simulink library "halin"  (R2021b)
settings: Solver=VariableStepAuto  StartTime=0.0  StopTime=10.0  RelTol=1e-3
undefined symbols (not defined in the file): TRUE
libraries: FVT_lib x100, hcu_lib x41
(part 9 of 10)

== system halin/HAL_IN/CAN3/MCU_B_R1/RrMCUErr ==
  Rr_MCUErr : Inport
  UnitConverter : DataTypeConversion  OutDataTypeStr=uint8
  VHAL_RrMCUErr_enum : Outport
  wires:
  UnitConverter/1 -> VHAL_RrMCUErr_enum/1
  Rr_MCUErr/1 -> UnitConverter/1

== system halin/HAL_IN/CAN3/MCU_B_R1/RrMCUIGNsta ==
  Rr_MCUIGN_sta : Inport
  UnitConverter : DataTypeConversion  OutDataTypeStr=uint8
  VHAL_RrMCUIGNsta_flg : Outport
  wires:
  UnitConverter/1 -> VHAL_RrMCUIGNsta_flg/1
  Rr_MCUIGN_sta/1 -> UnitConverter/1

== system halin/HAL_IN/CAN3/MCU_B_R1/RrMCUReady ==
  Rr_MCUReady : Inport
  UnitConverter : DataTypeConversion  OutDataTypeStr=uint8
  VHAL_RrMCUReady_flg : Outport
  wires:
  UnitConverter/1 -> VHAL_RrMCUReady_flg/1
  Rr_MCUReady/1 -> UnitConverter/1

== system halin/HAL_IN/CAN3/MCU_B_R1/RrMCUReady4Pre ==
  Rr_MCUReady4Pre : Inport
  UnitConverter : DataTypeConversion  OutDataTypeStr=uint8
  VHAL_RrMCUReady4Pre_flg : Outport
  wires:
  UnitConverter/1 -> VHAL_RrMCUReady4Pre_flg/1
  Rr_MCUReady4Pre/1 -> UnitConverter/1

== system halin/HAL_IN/CAN3/MCU_B_R1/RrMCUSysSta ==
  Rr_MCUSysSta : Inport
  UnitConverter : DataTypeConversion  OutDataTypeStr=uint8
  VHAL_RrMCUSysSta_enum : Outport
  wires:
  UnitConverter/1 -> VHAL_RrMCUSysSta_enum/1
  Rr_MCUSysSta/1 -> UnitConverter/1

== system halin/HAL_IN/CAN3/MCU_B_R1/RrMCUTemp ==
  Rr_MCUTemp : Inport
  UnitConverter : DataTypeConversion  OutDataTypeStr=uint16
  convert_in : FVT_lib/hal/convert_in  gain=1  offset=-40
  VHAL_RrMCUTemp_C : Outport
  wires:
  convert_in/1 -> VHAL_RrMCUTemp_C/1
  UnitConverter/1 -> convert_in/1
  Rr_MCUTemp/1 -> UnitConverter/1

== system halin/HAL_IN/CAN3/MCU_B_R1/RrMotorAvailTq ==
  Rr_MotorAvailTq : Inport
  UnitConverter : DataTypeConversion  OutDataTypeStr=uint16
  VHAL_RrMotorAvailTq_Nm : Outport
  wires:
  UnitConverter/1 -> VHAL_RrMotorAvailTq_Nm/1
  Rr_MotorAvailTq/1 -> UnitConverter/1

== system halin/HAL_IN/CAN3/MCU_B_R1/RrRegenAvailTq ==
  Rr_RegenAvailTq : Inport
  UnitConverter : DataTypeConversion  OutDataTypeStr=uint16
  convert_in : FVT_lib/hal/convert_in  gain=1  offset=-1022
  VHAL_RrRegenAvailTq_Nm : Outport
  wires:
  convert_in/1 -> VHAL_RrRegenAvailTq_Nm/1
  UnitConverter/1 -> convert_in/1
  Rr_RegenAvailTq/1 -> UnitConverter/1

== system halin/HAL_IN/CAN3/MCU_B_R1/RrTMSpd ==
  Rr_TMSpd : Inport
  UnitConverter : DataTypeConversion  OutDataTypeStr=uint16
  convert_in : FVT_lib/hal/convert_in  gain=1  offset=-18000
  VHAL_RrTMSpd_rpm : Outport
  wires:
  convert_in/1 -> VHAL_RrTMSpd_rpm/1
  UnitConverter/1 -> convert_in/1
  Rr_TMSpd/1 -> UnitConverter/1

== system halin/HAL_IN/CAN3/MCU_B_R1/RrTMTemp ==
  Rr_TMTemp : Inport
  UnitConverter : DataTypeConversion  OutDataTypeStr=uint16
  convert_in : FVT_lib/hal/convert_in  gain=1  offset=-40
  VHAL_RrTMTemp_C : Outport
  wires:
  convert_in/1 -> VHAL_RrTMTemp_C/1
  UnitConverter/1 -> convert_in/1
  Rr_TMTemp/1 -> UnitConverter/1

== system halin/HAL_IN/CAN3/MCU_B_R1/RrTMid ==
  Rr_TMid : Inport
  UnitConverter : DataTypeConversion  OutDataTypeStr=uint16
  convert_in : FVT_lib/hal/convert_in  gain=0.1  offset=-1500
  VHAL_RrTMid_A : Outport
  wires:
  convert_in/1 -> VHAL_RrTMid_A/1
  UnitConverter/1 -> convert_in/1
  Rr_TMid/1 -> UnitConverter/1

== system halin/HAL_IN/CAN3/MCU_B_R1/RrTMiq ==
  Rr_TMiq : Inport
  UnitConverter : DataTypeConversion  OutDataTypeStr=uint16
  convert_in : FVT_lib/hal/convert_in  gain=0.1  offset=-1500
  VHAL_RrTMiq_A : Outport
  wires:
  convert_in/1 -> VHAL_RrTMiq_A/1
  UnitConverter/1 -> convert_in/1
  Rr_TMiq/1 -> UnitConverter/1

== system halin/HAL_IN/CAN3/MCU_B_R2/RrCoolanttempReq ==
  Rr_CoolanttempReq : Inport
  UnitConverter : DataTypeConversion  OutDataTypeStr=uint16
  convert_in : FVT_lib/hal/convert_in  gain=1  offset=-40
  VHAL_RrCoolanttempReq_cnt : Outport
  wires:
  convert_in/1 -> VHAL_RrCoolanttempReq_cnt/1
  UnitConverter/1 -> convert_in/1
  Rr_CoolanttempReq/1 -> UnitConverter/1

== system halin/HAL_IN/CAN3/MCU_B_R2/RrFailcode1 ==
  Rr_Failcode1 : Inport
  UnitConverter : DataTypeConversion  OutDataTypeStr=uint8
  VHAL_RrFailcode1_enum : Outport
  wires:
  UnitConverter/1 -> VHAL_RrFailcode1_enum/1
  Rr_Failcode1/1 -> UnitConverter/1

== system halin/HAL_IN/CAN3/MCU_B_R2/RrFailcode2 ==
  Rr_Failcode2 : Inport
  UnitConverter : DataTypeConversion  OutDataTypeStr=uint8
  VHAL_RrFailcode2_enum : Outport
  wires:
  UnitConverter/1 -> VHAL_RrFailcode2_enum/1
  Rr_Failcode2/1 -> UnitConverter/1

== system halin/HAL_IN/CAN3/MCU_B_R2/RrFailcodehistory1 ==
  Rr_Failcodehistory1 : Inport
  UnitConverter : DataTypeConversion  OutDataTypeStr=uint8
  VHAL_RrFailcodehistory1_enum : Outport
  wires:
  UnitConverter/1 -> VHAL_RrFailcodehistory1_enum/1
  Rr_Failcodehistory1/1 -> UnitConverter/1

== system halin/HAL_IN/CAN3/MCU_B_R2/RrFailcodehistory2 ==
  Rr_Failcodehistory2 : Inport
  UnitConverter : DataTypeConversion  OutDataTypeStr=uint8
  VHAL_RrFailcodehistory2_enum : Outport
  wires:
  UnitConverter/1 -> VHAL_RrFailcodehistory2_enum/1
  Rr_Failcodehistory2/1 -> UnitConverter/1

== system halin/HAL_IN/CAN3/MCU_B_R2/RrLLCTemp ==
  Rr_LLCTemp : Inport
  UnitConverter : DataTypeConversion  OutDataTypeStr=uint16
  convert_in : FVT_lib/hal/convert_in  gain=1  offset=-40
  VHAL_RrLLCTemp_C : Outport
  wires:
  convert_in/1 -> VHAL_RrLLCTemp_C/1
  UnitConverter/1 -> convert_in/1
  Rr_LLCTemp/1 -> UnitConverter/1

== system halin/HAL_IN/CAN3/MCU_B_R2/RrLLCflowReq ==
  Rr_LLCflowReq : Inport
  UnitConverter : DataTypeConversion  OutDataTypeStr=uint8
  convert_in : FVT_lib/hal/convert_in  gain=0.25  offset=0
  VHAL_RrLLCflowReq_Lpmin : Outport
  wires:
  convert_in/1 -> VHAL_RrLLCflowReq_Lpmin/1
  UnitConverter/1 -> convert_in/1
  Rr_LLCflowReq/1 -> UnitConverter/1

== system halin/HAL_IN/CAN3/MCU_B_R2/RrMCU3HWVer ==
  Rr_MCU3_HW_Ver : Inport
  UnitConverter : DataTypeConversion  OutDataTypeStr=uint16
  VHAL_RrMCU3HWVer_enum : Outport
  wires:
  UnitConverter/1 -> VHAL_RrMCU3HWVer_enum/1
  Rr_MCU3_HW_Ver/1 -> UnitConverter/1

== system halin/HAL_IN/CAN3/MCU_B_R2/RrMCU3SWVer ==
  Rr_MCU3_SW_Ver : Inport
  UnitConverter : DataTypeConversion  OutDataTypeStr=uint16
  VHAL_RrMCU3SWVer_enum : Outport
  wires:
  UnitConverter/1 -> VHAL_RrMCU3SWVer_enum/1
  Rr_MCU3_SW_Ver/1 -> UnitConverter/1

== system halin/HAL_IN/CAN3/MCU_B_R2/RrMCUTempWarn ==
  Rr_MCUTempWarn : Inport
  UnitConverter : DataTypeConversion  OutDataTypeStr=uint8
  VHAL_RrMCUTempWarn_enum : Outport
  wires:
  UnitConverter/1 -> VHAL_RrMCUTempWarn_enum/1
  Rr_MCUTempWarn/1 -> UnitConverter/1

== system halin/HAL_IN/CAN3/MCU_B_R2/RrTMTempWarn ==
  Rr_TMTempWarn : Inport
  UnitConverter : DataTypeConversion  OutDataTypeStr=uint8
  VHAL_RrTMTempWarn_enum : Outport
  wires:
  UnitConverter/1 -> VHAL_RrTMTempWarn_enum/1
  Rr_TMTempWarn/1 -> UnitConverter/1

== system halin/HAL_IN/CAN3/Shifter1/ShifterCRC8 ==
  Shifter_CRC8 : Inport
  UnitConverter : DataTypeConversion  OutDataTypeStr=uint8
  VHAL_ShifterCRC8_enum : Outport
  wires:
  UnitConverter/1 -> VHAL_ShifterCRC8_enum/1
  Shifter_CRC8/1 -> UnitConverter/1

== system halin/HAL_IN/CAN3/Shifter1/ShifterFailsta ==
  Shifter_Fail_sta : Inport
  UnitConverter : DataTypeConversion  OutDataTypeStr=uint8
  VHAL_ShifterFailsta_enum : Outport
  wires:
  UnitConverter/1 -> VHAL_ShifterFailsta_enum/1
  Shifter_Fail_sta/1 -> UnitConverter/1

== system halin/HAL_IN/CAN3/Shifter1/ShifterHandleCmd ==
  Shifter_Handle_Cmd : Inport
  UnitConverter : DataTypeConversion  OutDataTypeStr=uint8
  VHAL_ShifterHandleCmd_enum : Outport
  wires:
  UnitConverter/1 -> VHAL_ShifterHandleCmd_enum/1
  Shifter_Handle_Cmd/1 -> UnitConverter/1

== system halin/HAL_IN/CAN3/Shifter1/ShifterRC ==
  Shifter_RC : Inport
  UnitConverter : DataTypeConversion  OutDataTypeStr=uint8
  VHAL_ShifterRC_enum : Outport
  wires:
  UnitConverter/1 -> VHAL_ShifterRC_enum/1
  Shifter_RC/1 -> UnitConverter/1

== system halin/HAL_IN/CAN4/DKC1/DKCReVehData ==
  DKC_Re_VehData : Inport
  UnitConverter : DataTypeConversion  OutDataTypeStr=uint8
  VHAL_DKCReVehData_enum : Outport
  wires:
  UnitConverter/1 -> VHAL_DKCReVehData_enum/1
  DKC_Re_VehData/1 -> UnitConverter/1

== system halin/HAL_IN/CAN4/DKC1/PCommandToBCM ==
  P_CommandToBCM : Inport
  UnitConverter : DataTypeConversion  OutDataTypeStr=uint8
  VHAL_PCommandToBCM_enum : Outport
  wires:
  UnitConverter/1 -> VHAL_PCommandToBCM_enum/1
  P_CommandToBCM/1 -> UnitConverter/1

== system halin/HAL_IN/CAN4/DKC1/PCommandToPTG ==
  P_CommandToPTG : Inport
  UnitConverter : DataTypeConversion  OutDataTypeStr=uint8
  VHAL_PCommandToPTG_enum : Outport
  wires:
  UnitConverter/1 -> VHAL_PCommandToPTG_enum/1
  P_CommandToPTG/1 -> UnitConverter/1

== system halin/HAL_IN/CAN4/DKC1/PDKeyAreaLockUnlock ==
  P_DKey_Area_LockUnlock : Inport
  UnitConverter : DataTypeConversion  OutDataTypeStr=uint8
  VHAL_PDKeyAreaLockUnlock_enum : Outport
  wires:
  UnitConverter/1 -> VHAL_PDKeyAreaLockUnlock_enum/1
  P_DKey_Area_LockUnlock/1 -> UnitConverter/1

== system halin/HAL_IN/CAN4/DKC1/PDKeyAreaPS ==
  P_DKey_Area_PS : Inport
  UnitConverter : DataTypeConversion  OutDataTypeStr=uint8
  VHAL_PDKeyAreaPS_enum : Outport
  wires:
  UnitConverter/1 -> VHAL_PDKeyAreaPS_enum/1
  P_DKey_Area_PS/1 -> UnitConverter/1

== system halin/HAL_IN/CAN4/DKC1/PDKeyAreaPTG ==
  P_DKey_Area_PTG : Inport
  UnitConverter : DataTypeConversion  OutDataTypeStr=uint8
  VHAL_PDKeyAreaPTG_enum : Outport
  wires:
  UnitConverter/1 -> VHAL_PDKeyAreaPTG_enum/1
  P_DKey_Area_PTG/1 -> UnitConverter/1

== system halin/HAL_IN/CAN4/DKC1/PDKeyWelcome ==
  P_DKey_Welcome : Inport
  UnitConverter : DataTypeConversion  OutDataTypeStr=uint8
  VHAL_PDKeyWelcome_enum : Outport
  wires:
  UnitConverter/1 -> VHAL_PDKeyWelcome_enum/1
  P_DKey_Welcome/1 -> UnitConverter/1

== system halin/HAL_IN/CAN4/DKC1/PDkeyShowIVI ==
  P_Dkey_Show_IVI : Inport
  UnitConverter : DataTypeConversion  OutDataTypeStr=uint8
  VHAL_PDkeyShowIVI_enum : Outport
  wires:
  UnitConverter/1 -> VHAL_PDkeyShowIVI_enum/1
  P_Dkey_Show_IVI/1 -> UnitConverter/1

== system halin/HAL_IN/CAN4/DKC1/PKeyMiss ==
  P_KeyMiss : Inport
  UnitConverter : DataTypeConversion  OutDataTypeStr=uint8
  VHAL_PKeyMiss_flg : Outport
  wires:
  UnitConverter/1 -> VHAL_PKeyMiss_flg/1
  P_KeyMiss/1 -> UnitConverter/1

== system halin/HAL_IN/CAN4/DKC1/PKeyMode ==
  P_KeyMode : Inport
  UnitConverter : DataTypeConversion  OutDataTypeStr=uint8
  VHAL_PKeyMode_enum : Outport
  wires:
  UnitConverter/1 -> VHAL_PKeyMode_enum/1
  P_KeyMode/1 -> UnitConverter/1

== system halin/HAL_IN/CAN4/DKC1/PUIDLowPower ==
  P_UID_LowPower : Inport
  UnitConverter : DataTypeConversion  OutDataTypeStr=uint8
  VHAL_PUIDLowPower_flg : Outport
  wires:
  UnitConverter/1 -> VHAL_PUIDLowPower_flg/1
  P_UID_LowPower/1 -> UnitConverter/1

== system halin/HAL_IN/CAN4/DKC2/EncryptionDATA063 ==
  EncryptionDATA_0_63 : Inport
  UnitConverter : DataTypeConversion  OutDataTypeStr=uint64
  VHAL_EncryptionDATA063_enum : Outport
  wires:
  UnitConverter/1 -> VHAL_EncryptionDATA063_enum/1
  EncryptionDATA_0_63/1 -> UnitConverter/1

== system halin/HAL_IN/CAN4/DKC2/EncryptionDATA64127 ==
  EncryptionDATA_64_127 : Inport
  UnitConverter : DataTypeConversion  OutDataTypeStr=uint64
  VHAL_EncryptionDATA64127_enum : Outport
  wires:
  UnitConverter/1 -> VHAL_EncryptionDATA64127_enum/1
  EncryptionDATA_64_127/1 -> UnitConverter/1

== system halin/HAL_IN/CAN4/DKC2/RandomNumberX ==
  Random_Number_X : Inport
  UnitConverter : DataTypeConversion  OutDataTypeStr=uint64
  VHAL_RandomNumberX_enum : Outport
  wires:
  UnitConverter/1 -> VHAL_RandomNumberX_enum/1
  Random_Number_X/1 -> UnitConverter/1

== system halin/HAL_IN/CAN4/Z24_C1000_0/Z24CHAAirPressureFC2Sta ==
  Z24_CHA_AirPressureFC2_Sta : Inport
  UnitConverter : DataTypeConversion  OutDataTypeStr=uint8
  convert_in : FVT_lib/hal/convert_in  gain=8  offset=0
  VHAL_Z24CHAAirPressureFC2Sta_KPa : Outport
  wires:
  convert_in/1 -> VHAL_Z24CHAAirPressureFC2Sta_KPa/1
  UnitConverter/1 -> convert_in/1
  Z24_CHA_AirPressureFC2_Sta/1 -> UnitConverter/1

== system halin/HAL_IN/CAN4/Z24_C1000_0/Z24CHAAirPressurePC3Sta ==
  Z24_CHA_AirPressurePC3_Sta : Inport
  UnitConverter : DataTypeConversion  OutDataTypeStr=uint8
  convert_in : FVT_lib/hal/convert_in  gain=8  offset=0
  VHAL_Z24CHAAirPressurePC3Sta_KPa : Outport
  wires:
  convert_in/1 -> VHAL_Z24CHAAirPressurePC3Sta_KPa/1
  UnitConverter/1 -> convert_in/1
  Z24_CHA_AirPressurePC3_Sta/1 -> UnitConverter/1

== system halin/HAL_IN/CAN4/Z24_C1000_0/Z24CHAAirPressureRC1Sta ==
  Z24_CHA_AirPressureRC1_Sta : Inport
  UnitConverter : DataTypeConversion  OutDataTypeStr=uint8
  convert_in : FVT_lib/hal/convert_in  gain=8  offset=0
  VHAL_Z24CHAAirPressureRC1Sta_KPa : Outport
  wires:
  convert_in/1 -> VHAL_Z24CHAAirPressureRC1Sta_KPa/1
  UnitConverter/1 -> convert_in/1
  Z24_CHA_AirPressureRC1_Sta/1 -> UnitConverter/1

== system halin/HAL_IN/CAN4/Z24_CE100_0/Z24BCMFWiperASSta ==
  Z24_BCM_FWiperAS_Sta : Inport
  UnitConverter : DataTypeConversion  OutDataTypeStr=uint8
  VHAL_Z24BCMFWiperASSta_flg : Outport
  wires:
  UnitConverter/1 -> VHAL_Z24BCMFWiperASSta_flg/1
  Z24_BCM_FWiperAS_Sta/1 -> UnitConverter/1

== system halin/HAL_IN/CAN4/Z24_CE100_0/Z24BCMSeatBeltSWSta ==
  Z24_BCM_SeatBeltSW_Sta : Inport
  UnitConverter : DataTypeConversion  OutDataTypeStr=uint8
  VHAL_Z24BCMSeatBeltSWSta_flg : Outport
  wires:
  UnitConverter/1 -> VHAL_Z24BCMSeatBeltSWSta_flg/1
  Z24_BCM_SeatBeltSW_Sta/1 -> UnitConverter/1

== system halin/HAL_IN/CAN4/ZONE_DR1/DrLockSta ==
  DrLockSta : Inport
  UnitConverter : DataTypeConversion  OutDataTypeStr=uint8
  VHAL_DrLockSta_flg : Outport
  wires:
  UnitConverter/1 -> VHAL_DrLockSta_flg/1
  DrLockSta/1 -> UnitConverter/1

== system halin/HAL_IN/CAN4/ZONE_DR1/MIRRORFOLDSW ==
  MIRROR_FOLD_SW : Inport
  UnitConverter : DataTypeConversion  OutDataTypeStr=uint8
  VHAL_MIRRORFOLDSW_flg : Outport
  wires:
  UnitConverter/1 -> VHAL_MIRRORFOLDSW_flg/1
  MIRROR_FOLD_SW/1 -> UnitConverter/1

== system halin/HAL_IN/CAN4/ZONE_DR1/RLTurnLampC ==
  RLTurnLampC : Inport
  UnitConverter : DataTypeConversion  OutDataTypeStr=uint8
  convert_in : FVT_lib/hal/convert_in  gain=10  offset=0
  VHAL_RLTurnLampC_mA : Outport
  wires:
  convert_in/1 -> VHAL_RLTurnLampC_mA/1
  UnitConverter/1 -> convert_in/1
  RLTurnLampC/1 -> UnitConverter/1

== system halin/HAL_IN/CAN4/ZONE_DR1/RRTurnLampC ==
  RRTurnLampC : Inport
  UnitConverter : DataTypeConversion  OutDataTypeStr=uint8
  convert_in : FVT_lib/hal/convert_in  gain=10  offset=0
  VHAL_RRTurnLampC_mA : Outport
  wires:
  convert_in/1 -> VHAL_RRTurnLampC_mA/1
  UnitConverter/1 -> convert_in/1
  RRTurnLampC/1 -> UnitConverter/1

== system halin/HAL_IN/CAN4/ZONE_DR1/RWiperAS ==
  RWiperAS : Inport
  UnitConverter : DataTypeConversion  OutDataTypeStr=uint8
  VHAL_RWiperAS_flg : Outport
  wires:
  UnitConverter/1 -> VHAL_RWiperAS_flg/1
  RWiperAS/1 -> UnitConverter/1

== system halin/HAL_IN/CAN4/ZONE_DR1/RWiperProtection ==
  RWiperProtection : Inport
  UnitConverter : DataTypeConversion  OutDataTypeStr=uint8
  VHAL_RWiperProtection_flg : Outport
  wires:
  UnitConverter/1 -> VHAL_RWiperProtection_flg/1
  RWiperProtection/1 -> UnitConverter/1

== system halin/HAL_IN/CAN4/ZONE_DR_VCU/BlowerErr ==
  Blower_Err : Inport
  UnitConverter : DataTypeConversion  OutDataTypeStr=uint8
  VHAL_BlowerErr_enum : Outport
  wires:
  UnitConverter/1 -> VHAL_BlowerErr_enum/1
  Blower_Err/1 -> UnitConverter/1

== system halin/HAL_IN/CAN4/ZONE_DR_VCU/DrPMMLVOutPErrLmp ==
  DrPMMLVOutPErrLmp : Inport
  UnitConverter : DataTypeConversion  OutDataTypeStr=uint8
  VHAL_DrPMMLVOutPErrLmp_flg : Outport
  wires:
  UnitConverter/1 -> VHAL_DrPMMLVOutPErrLmp_flg/1
  DrPMMLVOutPErrLmp/1 -> UnitConverter/1

== system halin/HAL_IN/CAN4/ZONE_DR_VCU/DrPMMSysErrLmp ==
  DrPMMSysErrLmp : Inport
  UnitConverter : DataTypeConversion  OutDataTypeStr=uint8
  VHAL_DrPMMSysErrLmp_flg : Outport
  wires:
  UnitConverter/1 -> VHAL_DrPMMSysErrLmp_flg/1
  DrPMMSysErrLmp/1 -> UnitConverter/1

== system halin/HAL_IN/CAN4/ZONE_DR_VCU/DrSCPSysErrLmp ==
  DrSCPSysErrLmp : Inport
  UnitConverter : DataTypeConversion  OutDataTypeStr=uint8
  VHAL_DrSCPSysErrLmp_flg : Outport
  wires:
  UnitConverter/1 -> VHAL_DrSCPSysErrLmp_flg/1
  DrSCPSysErrLmp/1 -> UnitConverter/1

== system halin/HAL_IN/CAN4/ZONE_DR_VCU/DrStdAErrSta ==
  DrStdAErrSta : Inport
  UnitConverter : DataTypeConversion  OutDataTypeStr=uint8
  VHAL_DrStdAErrSta_flg : Outport
  wires:
  UnitConverter/1 -> VHAL_DrStdAErrSta_flg/1
  DrStdAErrSta/1 -> UnitConverter/1

== system halin/HAL_IN/CAN4/ZONE_DR_VCU/SolarL ==
  SolarL : Inport
  UnitConverter : DataTypeConversion  OutDataTypeStr=uint8
  convert_in : FVT_lib/hal/convert_in  gain=5  offset=0
  VHAL_SolarL_W : Outport
  wires:
  convert_in/1 -> VHAL_SolarL_W/1
  UnitConverter/1 -> convert_in/1
  SolarL/1 -> UnitConverter/1

== system halin/HAL_IN/CAN4/ZONE_DR_VCU/SolarLErr ==
  SolarL_Err : Inport
  UnitConverter : DataTypeConversion  OutDataTypeStr=uint8
  VHAL_SolarLErr_enum : Outport
  wires:
  UnitConverter/1 -> VHAL_SolarLErr_enum/1
  SolarL_Err/1 -> UnitConverter/1

== system halin/HAL_IN/CAN4/ZONE_DR_VCU/SolarR ==
  SolarR : Inport
  UnitConverter : DataTypeConversion  OutDataTypeStr=uint8
  convert_in : FVT_lib/hal/convert_in  gain=5  offset=0
  VHAL_SolarR_W : Outport
  wires:
  convert_in/1 -> VHAL_SolarR_W/1
  UnitConverter/1 -> convert_in/1
  SolarR/1 -> UnitConverter/1

== system halin/HAL_IN/CAN4/ZONE_DR_VCU/SolarRErr ==
  SolarR_Err : Inport
  UnitConverter : DataTypeConversion  OutDataTypeStr=uint8
  VHAL_SolarRErr_enum : Outport
  wires:
  UnitConverter/1 -> VHAL_SolarRErr_enum/1
  SolarR_Err/1 -> UnitConverter/1

== system halin/HAL_IN/CAN4/ZONE_DR_VCU/TFaceL ==
  T_Face_L : Inport
  UnitConverter : DataTypeConversion  OutDataTypeStr=uint8
  convert_in : FVT_lib/hal/convert_in  gain=0.5  offset=-40
  VHAL_TFaceL_C : Outport
  wires:
  convert_in/1 -> VHAL_TFaceL_C/1
  UnitConverter/1 -> convert_in/1
  T_Face_L/1 -> UnitConverter/1

== system halin/HAL_IN/CAN4/ZONE_DR_VCU/TFaceLErr ==
  T_Face_L_Err : Inport
  UnitConverter : DataTypeConversion  OutDataTypeStr=uint8
  VHAL_TFaceLErr_enum : Outport
  wires:
  UnitConverter/1 -> VHAL_TFaceLErr_enum/1
  T_Face_L_Err/1 -> UnitConverter/1

== system halin/HAL_IN/CAN4/ZONE_DR_VCU/TFaceR ==
  T_Face_R : Inport
  UnitConverter : DataTypeConversion  OutDataTypeStr=uint8
  convert_in : FVT_lib/hal/convert_in  gain=0.5  offset=-40
  VHAL_TFaceR_C : Outport
  wires:
  convert_in/1 -> VHAL_TFaceR_C/1
  UnitConverter/1 -> convert_in/1
  T_Face_R/1 -> UnitConverter/1

== system halin/HAL_IN/CAN4/ZONE_DR_VCU/TFaceRErr ==
  T_Face_R_Err : Inport
  UnitConverter : DataTypeConversion  OutDataTypeStr=uint8
  VHAL_TFaceRErr_enum : Outport
  wires:
  UnitConverter/1 -> VHAL_TFaceRErr_enum/1
  T_Face_R_Err/1 -> UnitConverter/1

== system halin/HAL_IN/CAN4/ZONE_DR_VCU/TFaceRr ==
  T_Face_Rr : Inport
  UnitConverter : DataTypeConversion  OutDataTypeStr=uint8
  convert_in : FVT_lib/hal/convert_in  gain=0.5  offset=-40
  VHAL_TFaceRr_C : Outport
  wires:
  convert_in/1 -> VHAL_TFaceRr_C/1
  UnitConverter/1 -> convert_in/1
  T_Face_Rr/1 -> UnitConverter/1

== system halin/HAL_IN/CAN4/ZONE_DR_VCU/TFaceRrErr ==
  T_Face_Rr_Err : Inport
  UnitConverter : DataTypeConversion  OutDataTypeStr=uint8
  VHAL_TFaceRrErr_enum : Outport
  wires:
  UnitConverter/1 -> VHAL_TFaceRrErr_enum/1
  T_Face_Rr_Err/1 -> UnitConverter/1

== system halin/HAL_IN/CAN4/ZONE_DR_VCU/TFootL ==
  T_Foot_L : Inport
  UnitConverter : DataTypeConversion  OutDataTypeStr=uint8
  convert_in : FVT_lib/hal/convert_in  gain=0.5  offset=-40
  VHAL_TFootL_C : Outport
  wires:
  convert_in/1 -> VHAL_TFootL_C/1
  UnitConverter/1 -> convert_in/1
  T_Foot_L/1 -> UnitConverter/1

== system halin/HAL_IN/CAN4/ZONE_DR_VCU/TFootLErr ==
  T_Foot_L_Err : Inport
  UnitConverter : DataTypeConversion  OutDataTypeStr=uint8
  VHAL_TFootLErr_enum : Outport
  wires:
  UnitConverter/1 -> VHAL_TFootLErr_enum/1
  T_Foot_L_Err/1 -> UnitConverter/1

== system halin/HAL_IN/CAN4/ZONE_DR_VCU/TFootR ==
  T_Foot_R : Inport
  UnitConverter : DataTypeConversion  OutDataTypeStr=uint8
  convert_in : FVT_lib/hal/convert_in  gain=0.5  offset=-40
  VHAL_TFootR_C : Outport
  wires:
  convert_in/1 -> VHAL_TFootR_C/1
  UnitConverter/1 -> convert_in/1
  T_Foot_R/1 -> UnitConverter/1

== system halin/HAL_IN/CAN4/ZONE_DR_VCU/TFootRErr ==
  T_Foot_R_Err : Inport
  UnitConverter : DataTypeConversion  OutDataTypeStr=uint8
  VHAL_TFootRErr_enum : Outport
  wires:
  UnitConverter/1 -> VHAL_TFootRErr_enum/1
  T_Foot_R_Err/1 -> UnitConverter/1

== system halin/HAL_IN/CAN4/ZONE_DR_VCU/TFootRr ==
  T_Foot_Rr : Inport
  UnitConverter : DataTypeConversion  OutDataTypeStr=uint8
  convert_in : FVT_lib/hal/convert_in  gain=0.5  offset=-40
  VHAL_TFootRr_C : Outport
  wires:
  convert_in/1 -> VHAL_TFootRr_C/1
  UnitConverter/1 -> convert_in/1
  T_Foot_Rr/1 -> UnitConverter/1

== system halin/HAL_IN/CAN4/ZONE_DR_VCU/TFootRrErr ==
  T_Foot_Rr_Err : Inport
  UnitConverter : DataTypeConversion  OutDataTypeStr=uint8
  VHAL_TFootRrErr_enum : Outport
  wires:
  UnitConverter/1 -> VHAL_TFootRrErr_enum/1
  T_Foot_Rr_Err/1 -> UnitConverter/1

== system halin/HAL_IN/CAN4/ZONE_DR_VCU/Tevap ==
  Tevap : Inport
  UnitConverter : DataTypeConversion  OutDataTypeStr=uint8
  convert_in : FVT_lib/hal/convert_in  gain=0.5  offset=-40
  VHAL_Tevap_C : Outport
  wires:
  convert_in/1 -> VHAL_Tevap_C/1
  UnitConverter/1 -> convert_in/1
  Tevap/1 -> UnitConverter/1

== system halin/HAL_IN/CAN4/ZONE_DR_VCU/TevapErr ==
  Tevap_Err : Inport
  UnitConverter : DataTypeConversion  OutDataTypeStr=uint8
  VHAL_TevapErr_enum : Outport
  wires:
  UnitConverter/1 -> VHAL_TevapErr_enum/1
  Tevap_Err/1 -> UnitConverter/1

== system halin/HAL_IN/CAN4/ZONE_DR_VCU/Tincar ==
  Tincar : Inport
  UnitConverter : DataTypeConversion  OutDataTypeStr=uint8
  convert_in : FVT_lib/hal/convert_in  gain=0.5  offset=-40
  VHAL_Tincar_C : Outport
  wires:
  convert_in/1 -> VHAL_Tincar_C/1
  UnitConverter/1 -> convert_in/1
  Tincar/1 -> UnitConverter/1

== system halin/HAL_IN/CAN4/ZONE_DR_VCU/TincarErr ==
  Tincar_Err : Inport
  UnitConverter : DataTypeConversion  OutDataTypeStr=uint8
  VHAL_TincarErr_enum : Outport
  wires:
  UnitConverter/1 -> VHAL_TincarErr_enum/1
  Tincar_Err/1 -> UnitConverter/1

== system halin/HAL_IN/CAN4/ZONE_DR_VCU/ZoneDrMalfunLevel ==
  ZoneDrMalfunLevel : Inport
  UnitConverter : DataTypeConversion  OutDataTypeStr=uint8
  VHAL_ZoneDrMalfunLevel_enum : Outport
  wires:
  UnitConverter/1 -> VHAL_ZoneDrMalfunLevel_enum/1
  ZoneDrMalfunLevel/1 -> UnitConverter/1

== system halin/HAL_IN/CAN4/ZONE_FR1/ChargeInletLockSta ==
  ChargeInletLockSta : Inport
  UnitConverter : DataTypeConversion  OutDataTypeStr=uint8
  VHAL_ChargeInletLockSta_flg : Outport
  wires:
  UnitConverter/1 -> VHAL_ChargeInletLockSta_flg/1
  ChargeInletLockSta/1 -> UnitConverter/1

== system halin/HAL_IN/CAN4/ZONE_FR1/CompProEN ==
  CompProEN : Inport
  UnitConverter : DataTypeConversion  OutDataTypeStr=uint8
  VHAL_CompProEN_flg : Outport
  wires:
  UnitConverter/1 -> VHAL_CompProEN_flg/1
  CompProEN/1 -> UnitConverter/1

== system halin/HAL_IN/CAN4/ZONE_FR1/FLTurnLampC ==
  FLTurnLampC : Inport
  UnitConverter : DataTypeConversion  OutDataTypeStr=uint8
  convert_in : FVT_lib/hal/convert_in  gain=10  offset=0
  VHAL_FLTurnLampC_mA : Outport
  wires:
  convert_in/1 -> VHAL_FLTurnLampC_mA/1
  UnitConverter/1 -> convert_in/1
  FLTurnLampC/1 -> UnitConverter/1

== system halin/HAL_IN/CAN4/ZONE_FR1/FRTurnLampC ==
  FRTurnLampC : Inport
  UnitConverter : DataTypeConversion  OutDataTypeStr=uint8
  convert_in : FVT_lib/hal/convert_in  gain=10  offset=0
  VHAL_FRTurnLampC_mA : Outport
  wires:
  convert_in/1 -> VHAL_FRTurnLampC_mA/1
  UnitConverter/1 -> convert_in/1
  FRTurnLampC/1 -> UnitConverter/1

== system halin/HAL_IN/CAN4/ZONE_FR1/FWiperAS ==
  FWiperAS : Inport
  UnitConverter : DataTypeConversion  OutDataTypeStr=uint8
  VHAL_FWiperAS_flg : Outport
  wires:
  UnitConverter/1 -> VHAL_FWiperAS_flg/1
  FWiperAS/1 -> UnitConverter/1

== system halin/HAL_IN/CAN4/ZONE_FR1/FWiperProtection ==
  FWiperProtection : Inport
  UnitConverter : DataTypeConversion  OutDataTypeStr=uint8
  VHAL_FWiperProtection_flg : Outport
  wires:
  UnitConverter/1 -> VHAL_FWiperProtection_flg/1
  FWiperProtection/1 -> UnitConverter/1

== system halin/HAL_IN/CAN4/ZONE_FR1/TrailerCheck ==
  TrailerCheck : Inport
  UnitConverter : DataTypeConversion  OutDataTypeStr=uint8
  VHAL_TrailerCheck_flg : Outport
  wires:
  UnitConverter/1 -> VHAL_TrailerCheck_flg/1
  TrailerCheck/1 -> UnitConverter/1

== system halin/HAL_IN/CAN4/ZONE_FR1/TrailerModeSta ==
  TrailerModeSta : Inport
  UnitConverter : DataTypeConversion  OutDataTypeStr=uint8
  VHAL_TrailerModeSta_enum : Outport
  wires:
  UnitConverter/1 -> VHAL_TrailerModeSta_enum/1
  TrailerModeSta/1 -> UnitConverter/1

== system halin/HAL_IN/CAN4/ZONE_FR_VCU/BatInTemp ==
  Bat_In_Temp : Inport
  UnitConverter : DataTypeConversion  OutDataTypeStr=uint8
  convert_in : FVT_lib/hal/convert_in  gain=0.5  offset=-40
  VHAL_BatInTemp_C : Outport
  wires:
  convert_in/1 -> VHAL_BatInTemp_C/1
  UnitConverter/1 -> convert_in/1
  Bat_In_Temp/1 -> UnitConverter/1

== system halin/HAL_IN/CAN4/ZONE_FR_VCU/BatInTempErr ==
  Bat_In_Temp_Err : Inport
  UnitConverter : DataTypeConversion  OutDataTypeStr=uint8
  VHAL_BatInTempErr_enum : Outport
  wires:
  UnitConverter/1 -> VHAL_BatInTempErr_enum/1
  Bat_In_Temp_Err/1 -> UnitConverter/1

== system halin/HAL_IN/CAN4/ZONE_FR_VCU/BatOutTemp ==
  Bat_Out_Temp : Inport
  UnitConverter : DataTypeConversion  OutDataTypeStr=uint8
  convert_in : FVT_lib/hal/convert_in  gain=0.5  offset=-40
  VHAL_BatOutTemp_C : Outport
  wires:
  convert_in/1 -> VHAL_BatOutTemp_C/1
  UnitConverter/1 -> convert_in/1
  Bat_Out_Temp/1 -> UnitConverter/1

== system halin/HAL_IN/CAN4/ZONE_FR_VCU/COMPErr ==
  COMP_Err : Inport
  UnitConverter : DataTypeConversion  OutDataTypeStr=uint8
  VHAL_COMPErr_enum : Outport
  wires:
  UnitConverter/1 -> VHAL_COMPErr_enum/1
  COMP_Err/1 -> UnitConverter/1

== system halin/HAL_IN/CAN4/ZONE_FR_VCU/EACProtectEnable ==
  EACProtectEnable : Inport
  UnitConverter : DataTypeConversion  OutDataTypeStr=uint8
  VHAL_EACProtectEnable_enum : Outport
  wires:
  UnitConverter/1 -> VHAL_EACProtectEnable_enum/1
  EACProtectEnable/1 -> UnitConverter/1

== system halin/HAL_IN/CAN4/ZONE_FR_VCU/EWP3Err ==
  EWP3_Err : Inport
  UnitConverter : DataTypeConversion  OutDataTypeStr=uint8
  VHAL_EWP3Err_enum : Outport
  wires:
  UnitConverter/1 -> VHAL_EWP3Err_enum/1
  EWP3_Err/1 -> UnitConverter/1

== system halin/HAL_IN/CAN4/ZONE_FR_VCU/EXV1Err ==
  EXV1_Err : Inport
  UnitConverter : DataTypeConversion  OutDataTypeStr=uint8
  VHAL_EXV1Err_enum : Outport
  wires:
  UnitConverter/1 -> VHAL_EXV1Err_enum/1
  EXV1_Err/1 -> UnitConverter/1

== system halin/HAL_IN/CAN4/ZONE_FR_VCU/EXV2Err ==
  EXV2_Err : Inport
  UnitConverter : DataTypeConversion  OutDataTypeStr=uint8
  VHAL_EXV2Err_enum : Outport
  wires:
  UnitConverter/1 -> VHAL_EXV2Err_enum/1
  EXV2_Err/1 -> UnitConverter/1

== system halin/HAL_IN/CAN4/ZONE_FR_VCU/FanErr ==
  Fan_Err : Inport
  UnitConverter : DataTypeConversion  OutDataTypeStr=uint8
  VHAL_FanErr_enum : Outport
  wires:
  UnitConverter/1 -> VHAL_FanErr_enum/1
  Fan_Err/1 -> UnitConverter/1

== system halin/HAL_IN/CAN4/ZONE_FR_VCU/FrPMMLimpHomeActReq ==
  FrPMMLimpHomeActReq : Inport
  UnitConverter : DataTypeConversion  OutDataTypeStr=uint8
  VHAL_FrPMMLimpHomeActReq_flg : Outport
  wires:
  UnitConverter/1 -> VHAL_FrPMMLimpHomeActReq_flg/1
  FrPMMLimpHomeActReq/1 -> UnitConverter/1

== system halin/HAL_IN/CAN4/ZONE_FR_VCU/MotorInTemp ==
  Motor_In_Temp : Inport
  UnitConverter : DataTypeConversion  OutDataTypeStr=uint8
  convert_in : FVT_lib/hal/convert_in  gain=0.5  offset=-40
  VHAL_MotorInTemp_C : Outport
  wires:
  convert_in/1 -> VHAL_MotorInTemp_C/1
  UnitConverter/1 -> convert_in/1
  Motor_In_Temp/1 -> UnitConverter/1

== system halin/HAL_IN/CAN4/ZONE_FR_VCU/MotorInTempErr ==
  Motor_In_Temp_Err : Inport
  UnitConverter : DataTypeConversion  OutDataTypeStr=uint8
  VHAL_MotorInTempErr_enum : Outport
  wires:
  UnitConverter/1 -> VHAL_MotorInTempErr_enum/1
  Motor_In_Temp_Err/1 -> UnitConverter/1

== system halin/HAL_IN/CAN4/ZONE_FR_VCU/MotorOutTemp ==
  Motor_Out_Temp : Inport
  UnitConverter : DataTypeConversion  OutDataTypeStr=uint8
  convert_in : FVT_lib/hal/convert_in  gain=0.5  offset=-40
  VHAL_MotorOutTemp_C : Outport
  wires:
  convert_in/1 -> VHAL_MotorOutTemp_C/1
  UnitConverter/1 -> convert_in/1
  Motor_Out_Temp/1 -> UnitConverter/1

== system halin/HAL_IN/CAN4/ZONE_FR_VCU/MotorOutTempErr ==
  Motor_Out_Temp_Err : Inport
  UnitConverter : DataTypeConversion  OutDataTypeStr=uint8
  VHAL_MotorOutTempErr_enum : Outport
  wires:
  UnitConverter/1 -> VHAL_MotorOutTempErr_enum/1
  Motor_Out_Temp_Err/1 -> UnitConverter/1

== system halin/HAL_IN/CAN4/ZONE_FR_VCU/PTHighP ==
  PT_High_P : Inport
  UnitConverter : DataTypeConversion  OutDataTypeStr=uint16
  VHAL_PTHighP_KPa : Outport
  wires:
  UnitConverter/1 -> VHAL_PTHighP_KPa/1
  PT_High_P/1 -> UnitConverter/1

== system halin/HAL_IN/CAN4/ZONE_FR_VCU/PTHighPErr ==
  PT_High_P_Err : Inport
  UnitConverter : DataTypeConversion  OutDataTypeStr=uint8
  VHAL_PTHighPErr_enum : Outport
  wires:
  UnitConverter/1 -> VHAL_PTHighPErr_enum/1
  PT_High_P_Err/1 -> UnitConverter/1

== system halin/HAL_IN/CAN4/ZONE_FR_VCU/PTHighTact ==
  PT_High_Tact : Inport
  UnitConverter : DataTypeConversion  OutDataTypeStr=uint8
  convert_in : FVT_lib/hal/convert_in  gain=1  offset=-40
  VHAL_PTHighTact_C : Outport
  wires:
  convert_in/1 -> VHAL_PTHighTact_C/1
  UnitConverter/1 -> convert_in/1
  PT_High_Tact/1 -> UnitConverter/1

== system halin/HAL_IN/CAN4/ZONE_FR_VCU/PTHighTactErr ==
  PT_High_Tact_Err : Inport
  UnitConverter : DataTypeConversion  OutDataTypeStr=uint8
  VHAL_PTHighTactErr_enum : Outport
  wires:
  UnitConverter/1 -> VHAL_PTHighTactErr_enum/1
  PT_High_Tact_Err/1 -> UnitConverter/1

== system halin/HAL_IN/CAN4/ZONE_FR_VCU/PTLowP1 ==
  PT_Low_P1 : Inport
  UnitConverter : DataTypeConversion  OutDataTypeStr=uint16
  VHAL_PTLowP1_KPa : Outport
  wires:
  UnitConverter/1 -> VHAL_PTLowP1_KPa/1
  PT_Low_P1/1 -> UnitConverter/1

== system halin/HAL_IN/CAN4/ZONE_FR_VCU/PTLowP1Err ==
  PT_Low_P1_Err : Inport
  UnitConverter : DataTypeConversion  OutDataTypeStr=uint8
  VHAL_PTLowP1Err_enum : Outport
  wires:
  UnitConverter/1 -> VHAL_PTLowP1Err_enum/1
  PT_Low_P1_Err/1 -> UnitConverter/1

== system halin/HAL_IN/CAN4/ZONE_FR_VCU/PTLowP2 ==
  PT_Low_P2 : Inport
  UnitConverter : DataTypeConversion  OutDataTypeStr=uint16
  VHAL_PTLowP2_KPa : Outport
  wires:
  UnitConverter/1 -> VHAL_PTLowP2_KPa/1
  PT_Low_P2/1 -> UnitConverter/1

== system halin/HAL_IN/CAN4/ZONE_FR_VCU/PTLowP2Err ==
  PT_Low_P2_Err : Inport
  UnitConverter : DataTypeConversion  OutDataTypeStr=uint8
  VHAL_PTLowP2Err_enum : Outport
  wires:
  UnitConverter/1 -> VHAL_PTLowP2Err_enum/1
  PT_Low_P2_Err/1 -> UnitConverter/1

== system halin/HAL_IN/CAN4/ZONE_FR_VCU/PTLowT1 ==
  PT_Low_T1 : Inport
  UnitConverter : DataTypeConversion  OutDataTypeStr=uint8
  convert_in : FVT_lib/hal/convert_in  gain=0.5  offset=-40
  VHAL_PTLowT1_C : Outport
  wires:
  convert_in/1 -> VHAL_PTLowT1_C/1
  UnitConverter/1 -> convert_in/1
  PT_Low_T1/1 -> UnitConverter/1

== system halin/HAL_IN/CAN4/ZONE_FR_VCU/PTLowT1Err ==
  PT_Low_T1_Err : Inport
  UnitConverter : DataTypeConversion  OutDataTypeStr=uint8
  VHAL_PTLowT1Err_enum : Outport
  wires:
  UnitConverter/1 -> VHAL_PTLowT1Err_enum/1
  PT_Low_T1_Err/1 -> UnitConverter/1

== system halin/HAL_IN/CAN4/ZONE_FR_VCU/PTLowT2 ==
  PT_Low_T2 : Inport
  UnitConverter : DataTypeConversion  OutDataTypeStr=uint8
  convert_in : FVT_lib/hal/convert_in  gain=0.5  offset=-40
  VHAL_PTLowT2_C : Outport
  wires:
  convert_in/1 -> VHAL_PTLowT2_C/1
  UnitConverter/1 -> convert_in/1
  PT_Low_T2/1 -> UnitConverter/1

== system halin/HAL_IN/CAN4/ZONE_FR_VCU/PTLowT2Err ==
  PT_Low_T2_Err : Inport
  UnitConverter : DataTypeConversion  OutDataTypeStr=uint8
  VHAL_PTLowT2Err_enum : Outport
  wires:
  UnitConverter/1 -> VHAL_PTLowT2Err_enum/1
  PT_Low_T2_Err/1 -> UnitConverter/1

== system halin/HAL_IN/CAN4/ZONE_FR_VCU/SOTXVErr ==
  SOTXV_Err : Inport
  UnitConverter : DataTypeConversion  OutDataTypeStr=uint8
  VHAL_SOTXVErr_enum : Outport
  wires:
  UnitConverter/1 -> VHAL_SOTXVErr_enum/1
  SOTXV_Err/1 -> UnitConverter/1

== system halin/HAL_IN/CAN4/ZONE_FR_VCU/SOV1Err ==
  SOV1_Err : Inport
  UnitConverter : DataTypeConversion  OutDataTypeStr=uint8
  VHAL_SOV1Err_enum : Outport
  wires:
  UnitConverter/1 -> VHAL_SOV1Err_enum/1
  SOV1_Err/1 -> UnitConverter/1

== system halin/HAL_IN/CAN4/ZONE_FR_VCU/SOV2Err ==
  SOV2_Err : Inport
  UnitConverter : DataTypeConversion  OutDataTypeStr=uint8
  VHAL_SOV2Err_enum : Outport
  wires:
  UnitConverter/1 -> VHAL_SOV2Err_enum/1
  SOV2_Err/1 -> UnitConverter/1

== system halin/HAL_IN/CAN4/ZONE_FR_VCU/SOV3Err ==
  SOV3_Err : Inport
  UnitConverter : DataTypeConversion  OutDataTypeStr=uint8
  VHAL_SOV3Err_enum : Outport
  wires:
  UnitConverter/1 -> VHAL_SOV3Err_enum/1
  SOV3_Err/1 -> UnitConverter/1

== system halin/HAL_IN/CAN4/ZONE_FR_VCU/Tamb ==
  Tamb : Inport
  UnitConverter : DataTypeConversion  OutDataTypeStr=uint8
  convert_in : FVT_lib/hal/convert_in  gain=0.5  offset=-40
  VHAL_Tamb_C : Outport
  wires:
  convert_in/1 -> VHAL_Tamb_C/1
  UnitConverter/1 -> convert_in/1
  Tamb/1 -> UnitConverter/1

== system halin/HAL_IN/CAN4/ZONE_FR_VCU/TambErr ==
  Tamb_Err : Inport
  UnitConverter : DataTypeConversion  OutDataTypeStr=uint8
  VHAL_TambErr_enum : Outport
  wires:
  UnitConverter/1 -> VHAL_TambErr_enum/1
  Tamb_Err/1 -> UnitConverter/1

== system halin/HAL_IN/CAN4/zGW_APTC1/FrntPTCLeActHeatPwr ==
  FrntPTCLeActHeatPwr : Inport
  UnitConverter : DataTypeConversion  OutDataTypeStr=uint8
  convert_in : FVT_lib/hal/convert_in  gain=25  offset=0
  VHAL_FrntPTCLeActHeatPwr_W : Outport
  wires:
  convert_in/1 -> VHAL_FrntPTCLeActHeatPwr_W/1
  UnitConverter/1 -> convert_in/1
  FrntPTCLeActHeatPwr/1 -> UnitConverter/1

== system halin/HAL_IN/CAN4/zGW_APTC1/FrntPTCRearLeActHeatPwr ==
  FrntPTCRearLeActHeatPwr : Inport
  UnitConverter : DataTypeConversion  OutDataTypeStr=uint8
  convert_in : FVT_lib/hal/convert_in  gain=25  offset=0
  VHAL_FrntPTCRearLeActHeatPwr_W : Outport
  wires:
  convert_in/1 -> VHAL_FrntPTCRearLeActHeatPwr_W/1
  UnitConverter/1 -> convert_in/1
  FrntPTCRearLeActHeatPwr/1 -> UnitConverter/1

== system halin/HAL_IN/CAN4/zGW_APTC1/FrntPTCRearRiActHeatPwr ==
  FrntPTCRearRiActHeatPwr : Inport
  UnitConverter : DataTypeConversion  OutDataTypeStr=uint8
  convert_in : FVT_lib/hal/convert_in  gain=25  offset=0
  VHAL_FrntPTCRearRiActHeatPwr_W : Outport
  wires:
  convert_in/1 -> VHAL_FrntPTCRearRiActHeatPwr_W/1
  UnitConverter/1 -> convert_in/1
  FrntPTCRearRiActHeatPwr/1 -> UnitConverter/1

== system halin/HAL_IN/CAN4/zGW_APTC1/FrntPTCRiActHeatPwr ==
  FrntPTCRiActHeatPwr : Inport
  UnitConverter : DataTypeConversion  OutDataTypeStr=uint8
  convert_in : FVT_lib/hal/convert_in  gain=25  offset=0
  VHAL_FrntPTCRiActHeatPwr_W : Outport
  wires:
  convert_in/1 -> VHAL_FrntPTCRiActHeatPwr_W/1
  UnitConverter/1 -> convert_in/1
  FrntPTCRiActHeatPwr/1 -> UnitConverter/1

== system halin/HAL_IN/CAN4/zGW_CANFr1/COMPActualPwr ==
  COMP_ActualPwr : Inport
  UnitConverter : DataTypeConversion  OutDataTypeStr=uint16
  VHAL_COMPActualPwr_W : Outport
  wires:
  UnitConverter/1 -> VHAL_COMPActualPwr_W/1
  COMP_ActualPwr/1 -> UnitConverter/1

== system halin/HAL_IN/CAN4/zGW_CANFr1/COMPStatorSpd ==
  COMP_StatorSpd : Inport
  UnitConverter : DataTypeConversion  OutDataTypeStr=uint16
  VHAL_COMPStatorSpd_rpm : Outport
  wires:
  UnitConverter/1 -> VHAL_COMPStatorSpd_rpm/1
  COMP_StatorSpd/1 -> UnitConverter/1

== system halin/HAL_IN/CAN4/zGW_CANFr1/PTCActuPwrHSC6 ==
  PTCActuPwrHSC6 : Inport
  UnitConverter : DataTypeConversion  OutDataTypeStr=uint16
  VHAL_PTCActuPwrHSC6_enum : Outport
  wires:
  UnitConverter/1 -> VHAL_PTCActuPwrHSC6_enum/1
  PTCActuPwrHSC6/1 -> UnitConverter/1

== system halin/HAL_IN/CAN4/zGW_LINDr1/CSWDimSw ==
  CSW_DimSw : Inport
  UnitConverter : DataTypeConversion  OutDataTypeStr=uint8
  VHAL_CSWDimSw_flg : Outport
  wires:
  UnitConverter/1 -> VHAL_CSWDimSw_flg/1
  CSW_DimSw/1 -> UnitConverter/1

== system halin/HAL_IN/CAN4/zGW_LINDr1/CSWFWasSwSta ==
  CSW_FWasSw_Sta : Inport
  UnitConverter : DataTypeConversion  OutDataTypeStr=uint8
  VHAL_CSWFWasSwSta_enum : Outport
  wires:
  UnitConverter/1 -> VHAL_CSWFWasSwSta_enum/1
  CSW_FWasSw_Sta/1 -> UnitConverter/1

== system halin/HAL_IN/CAN4/zGW_LINDr1/CSWFWipSwSta ==
  CSW_FWipSw_Sta : Inport
  UnitConverter : DataTypeConversion  OutDataTypeStr=uint8
  VHAL_CSWFWipSwSta_enum : Outport
  wires:
  UnitConverter/1 -> VHAL_CSWFWipSwSta_enum/1
  CSW_FWipSw_Sta/1 -> UnitConverter/1

== system halin/HAL_IN/CAN4/zGW_LINDr1/CSWPassSWSta ==
  CSW_PassSW_Sta : Inport
  UnitConverter : DataTypeConversion  OutDataTypeStr=uint8
  VHAL_CSWPassSWSta_flg : Outport
  wires:
  UnitConverter/1 -> VHAL_CSWPassSWSta_flg/1
  CSW_PassSW_Sta/1 -> UnitConverter/1

== system halin/HAL_IN/CAN4/zGW_LINDr1/CSWRWasSWSta ==
  CSW_RWasSW_Sta : Inport
  UnitConverter : DataTypeConversion  OutDataTypeStr=uint8
  VHAL_CSWRWasSWSta_enum : Outport
  wires:
  UnitConverter/1 -> VHAL_CSWRWasSWSta_enum/1
  CSW_RWasSW_Sta/1 -> UnitConverter/1

== system halin/HAL_IN/CAN4/zGW_LINDr1/CSWRWipIntSwSta ==
  CSW_RWipIntSw_Sta : Inport
  UnitConverter : DataTypeConversion  OutDataTypeStr=uint8
  VHAL_CSWRWipIntSwSta_enum : Outport
  wires:
  UnitConverter/1 -> VHAL_CSWRWipIntSwSta_enum/1
  CSW_RWipIntSw_Sta/1 -> UnitConverter/1

== system halin/HAL_IN/CAN4/zGW_LINDr1/CSWTurnSwSta ==
  CSW_TurnSw_Sta : Inport
  UnitConverter : DataTypeConversion  OutDataTypeStr=uint8
  VHAL_CSWTurnSwSta_enum : Outport
  wires:
  UnitConverter/1 -> VHAL_CSWTurnSwSta_enum/1
  CSW_TurnSw_Sta/1 -> UnitConverter/1

== system halin/HAL_IN/CAN4/zGW_LINDr1/FAPWL01LINResponseError ==
  FAPWL_01_LIN_Response_Error : Inport
  UnitConverter : DataTypeConversion  OutDataTypeStr=uint8
  VHAL_FAPWL01LINResponseError_flg : Outport
  wires:
  UnitConverter/1 -> VHAL_FAPWL01LINResponseError_flg/1
  FAPWL_01_LIN_Response_Error/1 -> UnitConverter/1

== system halin/HAL_IN/CAN4/zGW_LINDr1/LDrvMotorRelayError ==
  L_Drv_Motor_Relay_Error : Inport
  UnitConverter : DataTypeConversion  OutDataTypeStr=uint8
  VHAL_LDrvMotorRelayError_flg : Outport
  wires:
  UnitConverter/1 -> VHAL_LDrvMotorRelayError_flg/1
  L_Drv_Motor_Relay_Error/1 -> UnitConverter/1

== system halin/HAL_IN/CAN4/zGW_LINDr1/LDrvMotorRippleError ==
  L_Drv_Motor_Ripple_Error : Inport
  UnitConverter : DataTypeConversion  OutDataTypeStr=uint8
  VHAL_LDrvMotorRippleError_flg : Outport
  wires:
  UnitConverter/1 -> VHAL_LDrvMotorRippleError_flg/1
  L_Drv_Motor_Ripple_Error/1 -> UnitConverter/1

== system halin/HAL_IN/CAN4/zGW_LINDr1/LDrvValWdwOpened ==
  L_Drv_Val_Wdw_Opened : Inport
  UnitConverter : DataTypeConversion  OutDataTypeStr=uint8
  VHAL_LDrvValWdwOpened_pct : Outport
  wires:
  UnitConverter/1 -> VHAL_LDrvValWdwOpened_pct/1
  L_Drv_Val_Wdw_Opened/1 -> UnitConverter/1

== system halin/HAL_IN/CAN4/zGW_LINDr1/LPasMotorRelayError ==
  L_Pas_Motor_Relay_Error : Inport
  UnitConverter : DataTypeConversion  OutDataTypeStr=uint8
  VHAL_LPasMotorRelayError_flg : Outport
  wires:
  UnitConverter/1 -> VHAL_LPasMotorRelayError_flg/1
  L_Pas_Motor_Relay_Error/1 -> UnitConverter/1

== system halin/HAL_IN/CAN4/zGW_LINDr1/LPasMotorRippleError ==
  L_Pas_Motor_Ripple_Error : Inport
  UnitConverter : DataTypeConversion  OutDataTypeStr=uint8
  VHAL_LPasMotorRippleError_flg : Outport
  wires:
  UnitConverter/1 -> VHAL_LPasMotorRippleError_flg/1
  L_Pas_Motor_Ripple_Error/1 -> UnitConverter/1

== system halin/HAL_IN/CAN4/zGW_LINDr1/LPasValWdwOpened ==
  L_Pas_Val_Wdw_Opened : Inport
  UnitConverter : DataTypeConversion  OutDataTypeStr=uint8
  VHAL_LPasValWdwOpened_pct : Outport
  wires:
  UnitConverter/1 -> VHAL_LPasValWdwOpened_pct/1
  L_Pas_Val_Wdw_Opened/1 -> UnitConverter/1

== system halin/HAL_IN/CAN4/zGW_LINDr1/LRLDMotorRelayError ==
  L_RLD_Motor_Relay_Error : Inport
  UnitConverter : DataTypeConversion  OutDataTypeStr=uint8
  VHAL_LRLDMotorRelayError_flg : Outport
  wires:
  UnitConverter/1 -> VHAL_LRLDMotorRelayError_flg/1
  L_RLD_Motor_Relay_Error/1 -> UnitConverter/1

== system halin/HAL_IN/CAN4/zGW_LINDr1/LRLDMotorRippleError ==
  L_RLD_Motor_Ripple_Error : Inport
  UnitConverter : DataTypeConversion  OutDataTypeStr=uint8
  VHAL_LRLDMotorRippleError_flg : Outport
  wires:
  UnitConverter/1 -> VHAL_LRLDMotorRippleError_flg/1
  L_RLD_Motor_Ripple_Error/1 -> UnitConverter/1

== system halin/HAL_IN/CAN4/zGW_LINDr1/LRLDValWdwOpened ==
  L_RLD_Val_Wdw_Opened : Inport
  UnitConverter : DataTypeConversion  OutDataTypeStr=uint8
  VHAL_LRLDValWdwOpened_pct : Outport
  wires:
  UnitConverter/1 -> VHAL_LRLDValWdwOpened_pct/1
  L_RLD_Val_Wdw_Opened/1 -> UnitConverter/1

== system halin/HAL_IN/CAN4/zGW_LINDr1/LRRDMotorRelayError ==
  L_RRD_Motor_Relay_Error : Inport
  UnitConverter : DataTypeConversion  OutDataTypeStr=uint8
  VHAL_LRRDMotorRelayError_flg : Outport
  wires:
  UnitConverter/1 -> VHAL_LRRDMotorRelayError_flg/1
  L_RRD_Motor_Relay_Error/1 -> UnitConverter/1

== system halin/HAL_IN/CAN4/zGW_LINDr1/LRRDMotorRippleError ==
  L_RRD_Motor_Ripple_Error : Inport
  UnitConverter : DataTypeConversion  OutDataTypeStr=uint8
  VHAL_LRRDMotorRippleError_flg : Outport
  wires:
  UnitConverter/1 -> VHAL_LRRDMotorRippleError_flg/1
  L_RRD_Motor_Ripple_Error/1 -> UnitConverter/1

== system halin/HAL_IN/CAN4/zGW_LINDr1/LRRDValWdwOpened ==
  L_RRD_Val_Wdw_Opened : Inport
  UnitConverter : DataTypeConversion  OutDataTypeStr=uint8
  VHAL_LRRDValWdwOpened_pct : Outport
  wires:
  UnitConverter/1 -> VHAL_LRRDValWdwOpened_pct/1
  L_RRD_Val_Wdw_Opened/1 -> UnitConverter/1

== system halin/HAL_IN/CAN4/zGW_LINDr1/RAPWL01LINResponseError ==
  RAPWL_01_LIN_Response_Error : Inport
  UnitConverter : DataTypeConversion  OutDataTypeStr=uint8
  VHAL_RAPWL01LINResponseError_flg : Outport
  wires:
  UnitConverter/1 -> VHAL_RAPWL01LINResponseError_flg/1
  RAPWL_01_LIN_Response_Error/1 -> UnitConverter/1

== system halin/HAL_IN/CAN4/zGW_LINDr1/RLSLampSta ==
  RLS_Lamp_Sta : Inport
  UnitConverter : DataTypeConversion  OutDataTypeStr=uint8
  VHAL_RLSLampSta_flg : Outport
  wires:
  UnitConverter/1 -> VHAL_RLSLampSta_flg/1
  RLS_Lamp_Sta/1 -> UnitConverter/1

== system halin/HAL_IN/CAN4/zGW_LINDr1/RLSRainSnrWiperCmd ==
  RLS_RainSnrWiperCmd : Inport
  UnitConverter : DataTypeConversion  OutDataTypeStr=uint8
  VHAL_RLSRainSnrWiperCmd_enum : Outport
  wires:
  UnitConverter/1 -> VHAL_RLSRainSnrWiperCmd_enum/1
  RLS_RainSnrWiperCmd/1 -> UnitConverter/1

== system halin/HAL_IN/CAN4/zGW_LINDr1/SWCACCSta ==
  SWC_ACC_Sta : Inport
  UnitConverter : DataTypeConversion  OutDataTypeStr=uint8
  VHAL_SWCACCSta_flg : Outport
  wires:
  UnitConverter/1 -> VHAL_SWCACCSta_flg/1
  SWC_ACC_Sta/1 -> UnitConverter/1

== system halin/HAL_IN/CAN4/zGW_LINDr1/SWCCANCELSta ==
  SWC_CANCEL_Sta : Inport
  UnitConverter : DataTypeConversion  OutDataTypeStr=uint8
  VHAL_SWCCANCELSta_flg : Outport
  wires:
  UnitConverter/1 -> VHAL_SWCCANCELSta_flg/1
  SWC_CANCEL_Sta/1 -> UnitConverter/1

== system halin/HAL_IN/CAN4/zGW_LINDr1/SWCDistanceSta ==
  SWC_Distance_Sta : Inport
  UnitConverter : DataTypeConversion  OutDataTypeStr=uint8
  VHAL_SWCDistanceSta_flg : Outport
  wires:
  UnitConverter/1 -> VHAL_SWCDistanceSta_flg/1
  SWC_Distance_Sta/1 -> UnitConverter/1

== system halin/HAL_IN/CAN4/zGW_LINDr1/SWCDownSta ==
  SWC_Down_Sta : Inport
  UnitConverter : DataTypeConversion  OutDataTypeStr=uint8
  VHAL_SWCDownSta_flg : Outport
  wires:
  UnitConverter/1 -> VHAL_SWCDownSta_flg/1
  SWC_Down_Sta/1 -> UnitConverter/1

== system halin/HAL_IN/CAN4/zGW_LINDr1/SWCLKASta ==
  SWC_LKA_Sta : Inport
  UnitConverter : DataTypeConversion  OutDataTypeStr=uint8
  VHAL_SWCLKASta_flg : Outport
  wires:
  UnitConverter/1 -> VHAL_SWCLKASta_flg/1
  SWC_LKA_Sta/1 -> UnitConverter/1

== system halin/HAL_IN/CAN4/zGW_LINDr1/SWCLeftSta ==
  SWC_Left_Sta : Inport
  UnitConverter : DataTypeConversion  OutDataTypeStr=uint8
  VHAL_SWCLeftSta_flg : Outport
  wires:
  UnitConverter/1 -> VHAL_SWCLeftSta_flg/1
  SWC_Left_Sta/1 -> UnitConverter/1

== system halin/HAL_IN/CAN4/zGW_LINDr1/SWCRegenUp ==
  SWC_RegenUp : Inport
  UnitConverter : DataTypeConversion  OutDataTypeStr=uint8
  VHAL_SWCRegenUp_flg : Outport
  wires:
  UnitConverter/1 -> VHAL_SWCRegenUp_flg/1
  SWC_RegenUp/1 -> UnitConverter/1

== system halin/HAL_IN/CAN4/zGW_LINDr1/SWCResUpSta ==
  SWC_Res_Up_Sta : Inport
  UnitConverter : DataTypeConversion  OutDataTypeStr=uint8
  VHAL_SWCResUpSta_flg : Outport
  wires:
  UnitConverter/1 -> VHAL_SWCResUpSta_flg/1
  SWC_Res_Up_Sta/1 -> UnitConverter/1

== system halin/HAL_IN/CAN4/zGW_LINDr1/SWCRightSta ==
  SWC_Right_Sta : Inport
  UnitConverter : DataTypeConversion  OutDataTypeStr=uint8
  VHAL_SWCRightSta_flg : Outport
  wires:
  UnitConverter/1 -> VHAL_SWCRightSta_flg/1
  SWC_Right_Sta/1 -> UnitConverter/1

== system halin/HAL_IN/CAN4/zGW_LINDr1/SWCSetdownSta ==
  SWC_Set_down_Sta : Inport
  UnitConverter : DataTypeConversion  OutDataTypeStr=uint8
  VHAL_SWCSetdownSta_flg : Outport
  wires:
  UnitConverter/1 -> VHAL_SWCSetdownSta_flg/1
  SWC_Set_down_Sta/1 -> UnitConverter/1

== system halin/HAL_IN/CAN4/zGW_LINDr1/SWCTripSta ==
  SWC_Trip_Sta : Inport
  UnitConverter : DataTypeConversion  OutDataTypeStr=uint8
  VHAL_SWCTripSta_flg : Outport
  wires:
  UnitConverter/1 -> VHAL_SWCTripSta_flg/1
  SWC_Trip_Sta/1 -> UnitConverter/1

== system halin/HAL_IN/CAN4/zGW_LINDr1/SWCUndefinedSta ==
  SWC_Undefined_Sta : Inport
  UnitConverter : DataTypeConversion  OutDataTypeStr=uint8
  VHAL_SWCUndefinedSta_flg : Outport
  wires:
  UnitConverter/1 -> VHAL_SWCUndefinedSta_flg/1
  SWC_Undefined_Sta/1 -> UnitConverter/1

== system halin/HAL_IN/CAN4/zGW_LINDr1/SWCUpSta ==
  SWC_Up_Sta : Inport
  UnitConverter : DataTypeConversion  OutDataTypeStr=uint8
  VHAL_SWCUpSta_flg : Outport
  wires:
  UnitConverter/1 -> VHAL_SWCUpSta_flg/1
  SWC_Up_Sta/1 -> UnitConverter/1

== system halin/HAL_IN/CAN4/zGW_LINDr1/SWCVRSta ==
  SWC_VR_Sta : Inport
  UnitConverter : DataTypeConversion  OutDataTypeStr=uint8
  VHAL_SWCVRSta_flg : Outport
  wires:
  UnitConverter/1 -> VHAL_SWCVRSta_flg/1
  SWC_VR_Sta/1 -> UnitConverter/1

== system halin/HAL_IN/CAN4/zGW_LINDr1/SWCmodeSta ==
  SWC_mode_Sta : Inport
  UnitConverter : DataTypeConversion  OutDataTypeStr=uint8
  VHAL_SWCmodeSta_flg : Outport
  wires:
  UnitConverter/1 -> VHAL_SWCmodeSta_flg/1
  SWC_mode_Sta/1 -> UnitConverter/1

== system halin/HAL_IN/CAN5/TBOX1/CbnPreACEnaReq ==
  CbnPreACEnaReq : Inport
  UnitConverter : DataTypeConversion  OutDataTypeStr=uint8
  VHAL_CbnPreACEnaReq_enum : Outport
  wires:
  UnitConverter/1 -> VHAL_CbnPreACEnaReq_enum/1
  CbnPreACEnaReq/1 -> UnitConverter/1

== system halin/HAL_IN/CAN5/TBOX1/PowerOffTSet ==
  PowerOff_T_Set : Inport
  UnitConverter : DataTypeConversion  OutDataTypeStr=uint8
  convert_in : FVT_lib/hal/convert_in  gain=1  offset=1
  VHAL_PowerOffTSet_cnt : Outport
  wires:
  convert_in/1 -> VHAL_PowerOffTSet_cnt/1
  UnitConverter/1 -> convert_in/1
  PowerOff_T_Set/1 -> UnitConverter/1

== system halin/HAL_IN/CAN5/TBOX1/ReDoorLock ==
  Re_DoorLock : Inport
  UnitConverter : DataTypeConversion  OutDataTypeStr=uint16
  VHAL_ReDoorLock_enum : Outport
  wires:
  UnitConverter/1 -> VHAL_ReDoorLock_enum/1
  Re_DoorLock/1 -> UnitConverter/1

== system halin/HAL_IN/CAN5/TBOX1/ReOutsideMirror ==
  ReOutsideMirror : Inport
  UnitConverter : DataTypeConversion  OutDataTypeStr=uint8
  VHAL_ReOutsideMirror_enum : Outport
  wires:
  UnitConverter/1 -> VHAL_ReOutsideMirror_enum/1
  ReOutsideMirror/1 -> UnitConverter/1

== system halin/HAL_IN/CAN5/TBOX1/RePwrReqTbox ==
  Re_PwrReqTbox : Inport
  UnitConverter : DataTypeConversion  OutDataTypeStr=uint8
  VHAL_RePwrReqTbox_enum : Outport
  wires:
  UnitConverter/1 -> VHAL_RePwrReqTbox_enum/1
  Re_PwrReqTbox/1 -> UnitConverter/1

== system halin/HAL_IN/CAN5/TBOX1/ReRadio ==
  Re_Radio : Inport
  UnitConverter : DataTypeConversion  OutDataTypeStr=uint8
  VHAL_ReRadio_flg : Outport
  wires:
  UnitConverter/1 -> VHAL_ReRadio_flg/1
  Re_Radio/1 -> UnitConverter/1

== system halin/HAL_IN/CAN5/TBOX1/RemoteACTemp ==
  Remote_ACTemp : Inport
  UnitConverter : DataTypeConversion  OutDataTypeStr=uint8
  convert_in : FVT_lib/hal/convert_in  gain=0.5  offset=17
  VHAL_RemoteACTemp_C : Outport
  wires:
  convert_in/1 -> VHAL_RemoteACTemp_C/1
  UnitConverter/1 -> convert_in/1
  Remote_ACTemp/1 -> UnitConverter/1

== system halin/HAL_IN/CAN5/TBOX1/RemoteAutoReq ==
  Remote_AutoReq : Inport
  UnitConverter : DataTypeConversion  OutDataTypeStr=uint8
  VHAL_RemoteAutoReq_flg : Outport
  wires:
  UnitConverter/1 -> VHAL_RemoteAutoReq_flg/1
  Remote_AutoReq/1 -> UnitConverter/1

== system halin/HAL_IN/CAN5/TBOX1/TBOXNETSIGSTR ==
  TBOX_NET_SIG_STR : Inport
  UnitConverter : DataTypeConversion  OutDataTypeStr=uint8
  VHAL_TBOXNETSIGSTR_enum : Outport
  wires:
  UnitConverter/1 -> VHAL_TBOXNETSIGSTR_enum/1
  TBOX_NET_SIG_STR/1 -> UnitConverter/1

== system halin/HAL_IN/CAN5/TBOX1/TBOXTESTSTATUS ==
  TBOX_TEST_STATUS : Inport
  UnitConverter : DataTypeConversion  OutDataTypeStr=uint8
  VHAL_TBOXTESTSTATUS_enum : Outport
  wires:
  UnitConverter/1 -> VHAL_TBOXTESTSTATUS_enum/1
  TBOX_TEST_STATUS/1 -> UnitConverter/1
